simulink model "dlbsTestHarnessAdam"  (R2025b)
settings: Solver=VariableStepAuto  StartTime=0.0  StopTime=10.0  RelTol=1e-3
undefined symbols (not defined in the file or in its folder): gamma
libraries: dlbsBlockAdam x1, dlbsBlockInsertGradientGF x1
settings Model: Creator=lt6037  LastModifiedBy=lt6037

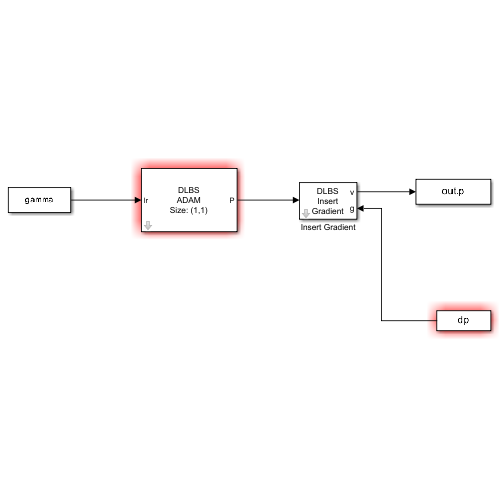
[thumbnail: Simulink's stored preview of the top-level diagram]
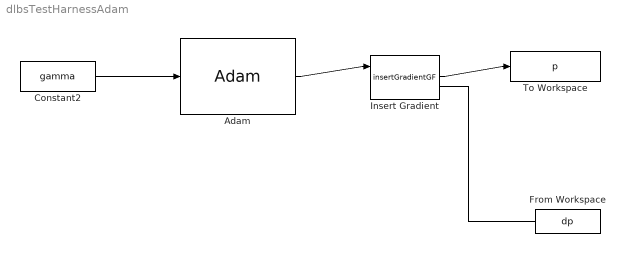
== system dlbsTestHarnessAdam ==
  Adam : dlbsBlockAdam/Adam  init=init  beta1=beta1  beta2=beta2  epsilon=epsilon
  Constant2 : Constant  Value=gamma  VectorParams1D=off
  From Workspace : FromWorkspace  VariableName=dp
  Insert Gradient : dlbsBlockInsertGradientGF/insertGradientGF
  To Workspace : ToWorkspace  VariableName=p  SaveFormat=Timeseries  SampleTime=-1
  wires:
  From Workspace/1 -> Insert Gradient/2
  Insert Gradient/1 -> To Workspace/1
  Constant2/1 -> Adam/1
  Adam/1 -> Insert Gradient/1
